simulink model "detect_change_test"  (Simulink 9.0)
settings: Solver=FixedStepDiscrete  StartTime=0.0  StopTime=10.0  FixedStep=0.200000  RelTol=1e-3  EnableMultiTasking=on
libraries: simulink x12
settings Model: SuppressorTable=22 serialization::archive 11 0 6 0 0 0 0 0  Creator=arnaud  LastModifiedBy=hbourbou
settings DataIOCC: LimitDataPoints=on  SaveFormat=StructureWithTime  SignalLoggingSaveFormat=ModelDataLogs
settings OptimizationCC: ExpressionDepthLimit=2147483647
settings DebuggingCC: SolverPrmCheckMsg=warning  FcnCallInpInsideContextMsg=warning  StateNameClashWarn=warning
settings GRTTargetCC: GeneratePreprocessorConditionals=Disable all  CombineOutputUpdateFcns=off  GRTInterface=on
settings ConfigComp: CovSFcnEnable=off

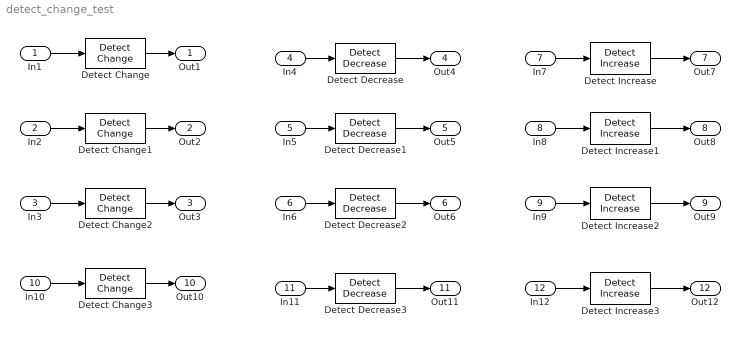
== system detect_change_test ==
  In1 : Inport  PortDimensions=1
  In2 : Inport  Port=2  PortDimensions=5
  In3 : Inport  Port=3  OutDataTypeStr=int8  PortDimensions=[2 3]
  In4 : Inport  Port=4  PortDimensions=1
  In5 : Inport  Port=5  PortDimensions=5
  In6 : Inport  Port=6  OutDataTypeStr=int8  PortDimensions=[2 3]
  In7 : Inport  Port=7  PortDimensions=1
  In8 : Inport  Port=8  PortDimensions=5
  In9 : Inport  Port=9  OutDataTypeStr=int8  PortDimensions=[2 3]
  In10 : Inport  Port=10  OutDataTypeStr=boolean  PortDimensions=1
  In11 : Inport  Port=11  OutDataTypeStr=boolean  PortDimensions=1
  In12 : Inport  Port=12  OutDataTypeStr=boolean  PortDimensions=1
  Detect Change{,1..3} (4 alike) : simulink/Logic and Bit Operations/Detect Change  vinit=0  InputProcessing=Inherited  OutDataTypeStr=boolean
  Detect Decrease{,1..3} (4 alike) : simulink/Logic and Bit Operations/Detect Decrease  vinit=0.0  InputProcessing=Inherited  OutDataTypeStr=boolean
  Detect Increase{,1..3} (4 alike) : simulink/Logic and Bit Operations/Detect Increase  vinit=0.0  InputProcessing=Inherited  OutDataTypeStr=boolean
  Out1 : Outport
  Out2 : Outport  Port=2
  Out3 : Outport  Port=3
  Out4 : Outport  Port=4
  Out5 : Outport  Port=5
  Out6 : Outport  Port=6
  Out7 : Outport  Port=7
  Out8 : Outport  Port=8
  Out9 : Outport  Port=9
  Out10 : Outport  Port=10
  Out11 : Outport  Port=11
  Out12 : Outport  Port=12
  wires:
  Detect Change/1 -> Out1/1
  In1/1 -> Detect Change/1
  Detect Change1/1 -> Out2/1
  In2/1 -> Detect Change1/1
  Detect Change2/1 -> Out3/1
  In3/1 -> Detect Change2/1
  In4/1 -> Detect Decrease/1
  In5/1 -> Detect Decrease1/1
  In6/1 -> Detect Decrease2/1
  In7/1 -> Detect Increase/1
  In8/1 -> Detect Increase1/1
  In9/1 -> Detect Increase2/1
  Detect Decrease/1 -> Out4/1
  Detect Decrease1/1 -> Out5/1
  Detect Decrease2/1 -> Out6/1
  Detect Increase/1 -> Out7/1
  Detect Increase1/1 -> Out8/1
  Detect Increase2/1 -> Out9/1
  Detect Change3/1 -> Out10/1
  In10/1 -> Detect Change3/1
  In11/1 -> Detect Decrease3/1
  In12/1 -> Detect Increase3/1
  Detect Decrease3/1 -> Out11/1
  Detect Increase3/1 -> Out12/1
